simulink model "matlab_actuator_model"  (R2015a)
settings: Solver=ode1  SolverMode=SingleTasking  StartTime=0.0  StopTime=100  FixedStep=0.1  MaxStep=0.1  RelTol=1e-3  AbsTol=1e-6
PreLoadFcn:
  | a1=3; a2=43;
PostLoadFcn:
  | optsiminit
settings Model: ExtModeTrigMode=oneshot  ExtModeArmWhenConnect=off  Creator=nikita  LastModifiedBy=vidigal
settings DataIOCC: LimitDataPoints=off  SignalLoggingSaveFormat=ModelDataLogs  SaveTime=off  StateSaveName=x  TimeSaveName=t
settings OptimizationCC: BooleanDataType=off  ExpressionDepthLimit=2147483647  InitFltsAndDblsToZero=on
settings DebuggingCC: SaveWithParameterizedLinksMsg=none  UnderspecifiedInitializationDetection=Classic  MergeDetectMultiDrivingBlocksExec=none  SignalResolutionControl=TryResolveAllWithWarning  MultiTaskDSMMsg=warning  MultiTaskCondExecSysMsg=none  IntegerOverflowMsg=none  FcnCallInpInsideContextMsg=UseLocalSettings  StateNameClashWarn=warning  IntegerSaturationMsg=none
settings HardwareCC: TargetUnknown=on
settings GRTTargetCC: TargetFcnLib=ansi_tfl_tmw.mat  CombineOutputUpdateFcns=off  GRTInterface=on

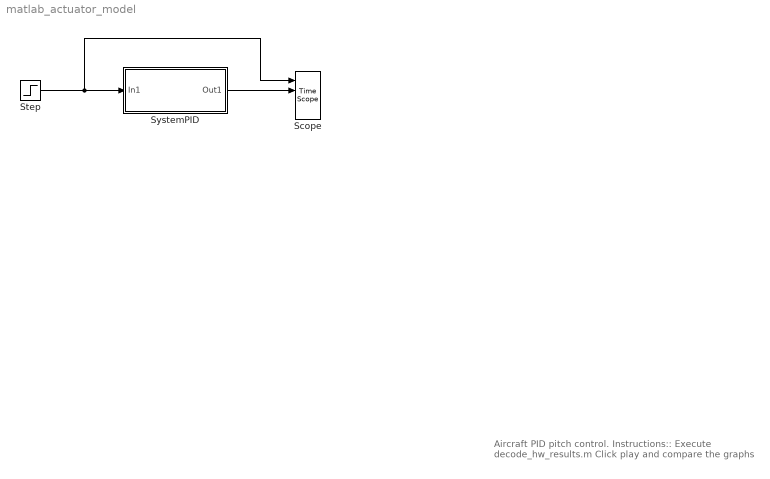
== system matlab_actuator_model ==
  note: Aircraft PID pitch control. Instructions::
      | Execute decode_hw_results.m
      | Click play and compare the graphs
  Scope : TimeScope  NumInputPorts=4
  Step : Step  Time=5  After=0.2  SampleTime=0.1
  SystemPID : Subsystem
  wires:
  Step/1 -> Scope/1, SystemPID/1(In1)
  SystemPID/1(Out1) -> Scope/2

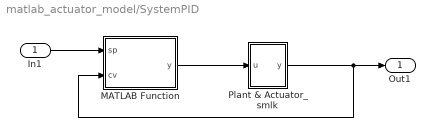
== system matlab_actuator_model/SystemPID ==
  In1 : Inport
  MATLAB Function : MATLAB Function
  Plant & Actuator_smlk : Subsystem
  Out1 : Outport
  wires:
  MATLAB Function/1(y) -> Plant & Actuator_smlk/1("u ")
  Plant & Actuator_smlk/1(y) -> Out1/1, MATLAB Function/2(cv)
  In1/1 -> MATLAB Function/1(sp)

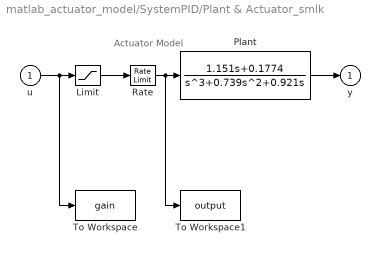
== system matlab_actuator_model/SystemPID/Plant & Actuator_smlk ==
  note: Actuator Model
  "u " : Inport
  Limit : Saturate  UpperLimit=2  LowerLimit=-2
  Plant : TransferFcn  Numerator=[1.151 0.1774]  Denominator=[1 0.739 0.921 0]
  Rate : RateLimiter  RisingSlewLimit=0.8  FallingSlewLimit=-0.8
  To Workspace : ToWorkspace  VariableName=gain  SaveFormat=Timeseries  SampleTime=-1
  To Workspace1 : ToWorkspace  VariableName=output  SaveFormat=Timeseries  SampleTime=-1
  y : Outport  InitialOutput=0
  wires:
  Plant/1 -> y/1
  "u "/1 -> To Workspace/1, Limit/1
  Limit/1 -> Rate/1
  Rate/1 -> To Workspace1/1, Plant/1

== matlab function matlab_actuator_model/SystemPID/MATLAB Function ==
  data: sp input; y output; cv input
% Aircraft Pich Control Example
% Introducing TMR for fault tolerance capabilities
% Daniel M. Munoz
% UnB and KTH
% March 2016

% For a step reference of 0.2 radians, the design criteria are the following.
% 1. Overshoot less than 10%
% 2. Rise time less than 2 seconds
% 3. Settling time less than 10 seconds
% 4. Steady-state error less than 2%

function y = fcn(sp,cv)

kp = 0.578125;
tad_i = 0.9375;
td_ad = 0.8125;
e_n_1 = 0;

ki = kp*tad_i;
kd = kp*td_ad;

e_n = sp - cv;
if sp == 0
    c = 0;
else
    c = kp*e_n + ki*(e_n+e_n_1) + kd*(e_n-e_n_1);
    e_n_1 = e_n;
end

y = c;
